simulink model "abEPMAFPLL_compare_sim_c"  (R2020b)
settings: Solver=FixedStepAuto  StartTime=0.0  StopTime=11  FixedStep=Ts  MaxStep=1e-5  RelTol=1e-3
undefined symbols (not defined in the file or in its folder): A_frq_step, A_phase_step, DiscIntNeverNeededParam, f_rad, k_phi, ki, kp, N, t_frq_step, t_phase_step, Ts, V_g, var_noise
libraries: simulink x9, bach_library x3
settings Model: Creator=Martin  LastModifiedBy=Kasper Laustsen
settings DataIOCC: ExternalInput=tt1, tt2, tt3, tt4, tt5, tt6  LoadExternalInput=on
settings SFSimCC: SimCustomHeaderCode=|
  | #include "PLL.h"
  | #include "MAF.h"
settings SFSimCC: SimUserSources=|
  | PLL.c
  | MAF.c

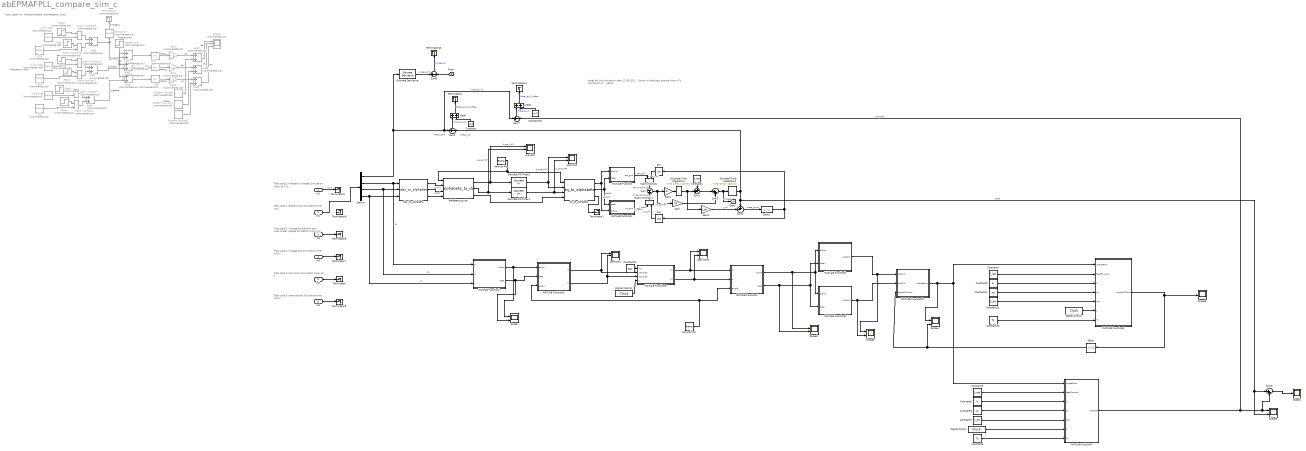
== system abEPMAFPLL_compare_sim_c ==
  note: Input signal incl. noise and phase- and frequency jump
  note: Notes for this simulation
      |
      | date: 22-03-2021,
      | - Solver is fixed step, sample time is Ts (constants.m) - 10kHz
  note: Noise
  note: Phase-jump
  note: theta_grid
  note: theta_pll
  note: Frequency-jump
  note: Test case 2: Phase jumps
      | Simulation time: 70 s
  note: Test case 1: Frequency changes
      | Simulation time: 36.72 s
  note: Test case 3: Voltage fluctuations
      | and over-/under voltage
      | Simulation time: 70 s
  note: Test case 4: Voltage dips
      | Simulation time: 40.9 s
  note: Test case 5: Harmonics
      | Simulation time: 40 s
  note: Test case 6: Interruptions
      | Simulation time: 40.6 s
  In1 : Inport  PortDimensions=4
  In2 : Inport  Port=2  PortDimensions=4
  In3 : Inport  Port=3  PortDimensions=4
  In4 : Inport  Port=4  PortDimensions=4
  In5 : Inport  Port=5  PortDimensions=4
  In6 : Inport  Port=6  PortDimensions=4
  Add{,1..5,7..9} (9 alike) : Sum  Commented=on
  Add11 : Sum
  Add6 : Sum
  Constant : Constant  Value=-pi/2
  Constant1 : Constant  Value=f_rad
  Constant10 : Constant  Value=Ts
  Constant11 : Constant  Value=kp
  Constant12 : Constant  Value=k_phi
  Constant13 : Constant  Value=-pi/2
  Constant24 : Constant  Value=200
  Constant3 : Constant  Value=f_rad
  Constant4 : Constant  Value=f_rad
  Constant5 : Constant  Value=ki
  Constant6 : Constant  Value=kp
  Constant7 : Constant  Value=k_phi
  Constant8 : Constant  Value=Ts
  Constant9 : Constant  Value=ki
  Cos : Trigonometry  Operator=cos
  Delay : Delay  DelayLength=1  SampleTime=Ts
  Delay1 : Delay  DelayLength=1
  Demux : Demux
  Derivative : Derivative  Commented=on
  Digital Clock1 : DigitalClock  SampleTime=Ts
  Digital Clock10 : DigitalClock  SampleTime=Ts
  Digital Clock2 : DigitalClock  SampleTime=Ts
  Discrete Derivative : simulink/Discrete/Discrete Derivative  gainval=1.0  ICPrevScaledInput=0.0  OutMin=[]  OutMax=[]  OutDataType=fixdt(1, 16)  OutScaling=2^-10  DoSatur=off
  Discrete FIR Filter1 : DiscreteFir  Coefficients=[ones(1,N).*1/N]
  Discrete FIR Filter3 : DiscreteFir  Coefficients=[ones(1,N).*1/N]
  Discrete-Time Integrator1 : DiscreteIntegrator  IntegratorMethod=Integration: Trapezoidal  SampleTime=-1  ICPrevOutput=DiscIntNeverNeededParam  ICPrevScaledInput=DiscIntNeverNeededParam
  Discrete-Time Integrator2 : DiscreteIntegrator  IntegratorMethod=Integration: Trapezoidal  SampleTime=-1  ICPrevOutput=DiscIntNeverNeededParam  ICPrevScaledInput=DiscIntNeverNeededParam
  Gain : Gain  Gain=kp
  Gain1 : Gain  Gain=ki
  Gain2 : Gain  Gain=k_phi
  Gain3 : Gain  Commented=on  Gain=V_g
  Gain4 : Gain  Commented=on  Gain=V_g
  Gain5 : Gain  Commented=on  Gain=V_g
  MATLAB Function : MATLAB Function  TreatAsAtomicUnit=on
  MATLAB Function1 : MATLAB Function  TreatAsAtomicUnit=on
  MATLAB Function10 : MATLAB Function  TreatAsAtomicUnit=on
  MATLAB Function2 : MATLAB Function  TreatAsAtomicUnit=on
  MATLAB Function3 : MATLAB Function  TreatAsAtomicUnit=on
  MATLAB Function4 : MATLAB Function  TreatAsAtomicUnit=on
  MATLAB Function5 : MATLAB Function  TreatAsAtomicUnit=on
  MATLAB Function6 : MATLAB Function  TreatAsAtomicUnit=on
  MATLAB Function7 : MATLAB Function  TreatAsAtomicUnit=on
  MATLAB Function8 : MATLAB Function  TreatAsAtomicUnit=on
  MATLAB Function9 : MATLAB Function  TreatAsAtomicUnit=on
  Matrix Multiply : Product
  Matrix Multiply1 : Product
  Matrix Multiply{2..7} (6 alike) : Product  Commented=on
  Random Number : RandomNumber  Commented=on  Variance=var_noise
  Random Number1 : RandomNumber  Commented=on  Variance=var_noise  Seed=1
  Random Number2 : RandomNumber  Commented=on  Variance=var_noise  Seed=2
  Scope{,2..5} (5 alike) : Scope  NumInputPorts=2
  Scope1 : Scope
  Scope6 : Scope
  Sin : Trigonometry
  Sin3 : Trigonometry  Commented=on
  Sin4 : Trigonometry  Commented=on
  Sin5 : Trigonometry  Commented=on
  Step : Step  Commented=on  Time=t_frq_step  Before=1  After=0  SampleTime=0
  Step1 : Step  Commented=on  Time=t_frq_step  SampleTime=0
  Step2 : Step  Commented=on  Time=t_frq_step  Before=1  After=0  SampleTime=0
  Step3 : Step  Commented=on  Time=t_frq_step  SampleTime=0
  Step4 : Step  Commented=on  Time=t_frq_step  Before=1  After=0  SampleTime=0
  Step5 : Step  Commented=on  Time=t_frq_step  SampleTime=0
  Sum : Sum  Inputs=-|+
  Sum1 : Sum  Inputs=++|
  Sum2 : Sum  Inputs=+|-
  Sum3 : Sum  Inputs=|++
  Sum4 : Sum  Inputs=+-|
  Sum6 : Sum  Inputs=+|-
  Sum7 : Sum  Inputs=+|-
  Sum8 : Sum  Inputs=|+-
  Terminator{,1..2,5..11} (10 alike) : Terminator
  Terminator3 : Terminator  Commented=on
  a_frq : simulink/Sources/Ramp  Commented=on  slope=f_rad  start=0  InitialOutput=0
  a_frq_step : simulink/Sources/Ramp  Commented=on  slope=f_rad*A_frq_step  start=t_frq_step  InitialOutput=t_frq_step*f_rad
  abc_to_alphabeta : bach_library/abc_to_alphabeta  SystemSampleTime=-1  VariantActivationTime=update diagram  Latency=0  AutoFrameSizeCalculation=off
  alphabeta_to_dq : bach_library/alphabeta_to_dq  SystemSampleTime=-1  VariantActivationTime=update diagram  Latency=0  AutoFrameSizeCalculation=off
  b_frq : simulink/Sources/Ramp  Commented=on  slope=f_rad  start=0  InitialOutput=-pi*2/3
  b_frq_step : simulink/Sources/Ramp  Commented=on  slope=f_rad*A_frq_step  start=t_frq_step  InitialOutput=t_frq_step*f_rad-pi*2/3
  c_frq : simulink/Sources/Ramp  Commented=on  slope=f_rad  start=0  InitialOutput=pi*2/3
  c_frq_step : simulink/Sources/Ramp  Commented=on  slope=f_rad*A_frq_step  start=t_frq_step  InitialOutput=t_frq_step*f_rad+pi*2/3
  dq_to_alphabeta : bach_library/dq_to_alphabeta  SystemSampleTime=-1  VariantActivationTime=update diagram  Latency=0  AutoFrameSizeCalculation=off
  nominal frq : simulink/Sources/Ramp  slope=f_rad  start=0  InitialOutput=0
  nominal frq1 : simulink/Sources/Ramp  slope=f_rad  start=0  InitialOutput=0
  phase-jump : Step  Commented=on  Time=t_phase_step  After=A_phase_step  SampleTime=0
  phases : Scope  Commented=on  NumInputPorts=3
  post MAF : Scope  NumInputPorts=2
  post MAF1 : Scope  NumInputPorts=2
  pre MAF : Scope  NumInputPorts=3
  pre MAF1 : Scope  NumInputPorts=3
  wires:
  Derivative/1 -> Terminator3/1  "omega_g"
  Step2/1 -> Matrix Multiply2/1
  MATLAB Function/1(cos_grid) -> Matrix Multiply/1  "cos_grid"
  Constant/1 -> Add6/2
  Step/1 -> Matrix Multiply5/1
  Sin5/1 -> Gain5/1  "theta_g"
  Sin3/1 -> Gain3/1  "theta_g"
  Step1/1 -> Matrix Multiply6/1
  a_frq/1 -> Matrix Multiply5/2
  Step4/1 -> Matrix Multiply4/1
  Matrix Multiply2/1 -> Add4/2
  Matrix Multiply7/1 -> Add5/1
  Matrix Multiply6/1 -> Add3/1
  a_frq_step/1 -> Matrix Multiply6/2
  Add6/1 -> Terminator2/1  "theta_err_sim_offset"
  Sum2/1 -> Add6/1  "theta_err_sim"
  Sin/1 -> Matrix Multiply/2  "sin_pll"
  Add1/1 -> Sin4/1
  phase-jump/1 -> Add/1, Add2/1, Add1/1
  Matrix Multiply4/1 -> Add5/2
  Add4/1 -> Add1/2  "b_phase"
  Add9/1 -> phases/3  "pc"
  Add5/1 -> Add2/2  "c_phase"
  Cos/1 -> Matrix Multiply1/2  "cos_pll"
  Add7/1 -> phases/1  "pa"
  Matrix Multiply/1 -> Sum/1  "cos_grid_sin_pll"
  Add8/1 -> phases/2  "pb"
  Add/1 -> Sin3/1
  Random Number/1 -> Add7/2
  Step3/1 -> Matrix Multiply3/1
  Add2/1 -> Sin5/1
  Gain3/1 -> Add7/1  "pa"
  c_frq/1 -> Matrix Multiply4/2
  Matrix Multiply5/1 -> Add3/2
  Add3/1 -> Add/2, Derivative/1  "a_phase"
  Matrix Multiply3/1 -> Add4/1
  Sin4/1 -> Gain4/1  "theta_g"
  MATLAB Function1/1(sin_grid) -> Matrix Multiply1/1  "sin_grid"
  Matrix Multiply1/1 -> Sum/2  "sin_grid_cos_pll"
  Random Number1/1 -> Add8/2
  b_frq_step/1 -> Matrix Multiply3/2
  Random Number2/1 -> Add9/2
  b_frq/1 -> Matrix Multiply2/2
  c_frq_step/1 -> Matrix Multiply7/2
  Gain5/1 -> Add9/1  "pc"
  Gain4/1 -> Add8/1  "pb"
  Step5/1 -> Matrix Multiply7/1
  Gain1/1 -> Discrete-Time Integrator1/1
  Gain/1 -> Sum3/2
  Discrete-Time Integrator1/1 -> Sum1/2, Gain2/1
  Discrete-Time Integrator2/1 -> Scope5/2, Sum8/1, Sum4/1, Sum2/2  "theta"
  Gain2/1 -> Sum4/2  "k_phi"
  Sum4/1 -> Delay1/1  "theta_comp"
  abc_to_alphabeta/3 -> alphabeta_to_dq/4
  dq_to_alphabeta/1 -> MATLAB Function/1(alpha), MATLAB Function1/2(alpha)  "alpha2"
  dq_to_alphabeta/2 -> MATLAB Function1/1(beta), MATLAB Function/2(beta)  "beta2"
  nominal frq/1 -> dq_to_alphabeta/1, alphabeta_to_dq/1
  abc_to_alphabeta/1 -> alphabeta_to_dq/2  "alpha1"
  abc_to_alphabeta/2 -> alphabeta_to_dq/3  "beta1"
  alphabeta_to_dq/2 -> Discrete FIR Filter1/1, pre MAF/2  "q_pre_MAF"
  alphabeta_to_dq/1 -> pre MAF/1, Discrete FIR Filter3/1  "d_pre_MAF"
  Discrete FIR Filter3/1 -> post MAF/1, dq_to_alphabeta/2  "d_post_MAF"
  Discrete FIR Filter1/1 -> post MAF/2, dq_to_alphabeta/3  "q_post_MAF"
  alphabeta_to_dq/3 -> dq_to_alphabeta/4
  Sum1/1 -> Sum3/1
  Constant1/1 -> Sum1/1
  Sum3/1 -> Discrete-Time Integrator2/1, [A]  "omega"
  dq_to_alphabeta/3 -> Terminator1/1
  Demux/1 -> Sum7/1, Sum2/1, Discrete Derivative/1  "thetha_hilb"
  Discrete Derivative/1 -> Sum6/1  "omega_hilb"
  [A] -> Sum6/2
  Sum6/1 -> Terminator10/1  "omega_err"
  In1/1 -> Terminator5/1  "Input"
  In2/1 -> Demux/1
  In3/1 -> Terminator6/1
  In4/1 -> Terminator7/1
  In5/1 -> Terminator/1
  In6/1 -> Terminator8/1
  Sum/1 -> Gain1/1, Gain/1  "sin_grid-pll"
  MATLAB Function9/1(y1) -> post MAF1/1, MATLAB Function4/1(d)
  MATLAB Function9/2(y2) -> post MAF1/2, MATLAB Function4/2(q)
  MATLAB Function3/1(d) -> pre MAF1/1, MATLAB Function9/2(sample1)
  Constant24/1 -> MATLAB Function9/1(len)
  nominal frq1/1 -> MATLAB Function3/3(angle), MATLAB Function4/3(angle)
  MATLAB Function3/2(q) -> pre MAF1/2, MATLAB Function9/3(sample2)
  Delay/1 -> Scope4/2, MATLAB Function10/3(anglePllComp)
  Constant7/1 -> MATLAB Function7/5(kPhi)
  MATLAB Function10/1(phaseError) -> Scope4/1, MATLAB Function7/1(phaseError), MATLAB Function8/1(phaseError)
  MATLAB Function2/1(alpha) -> Scope/1, MATLAB Function3/1(alpha)
  Constant11/1 -> MATLAB Function8/4(kp)
  Constant6/1 -> MATLAB Function7/4(kp)
  Constant9/1 -> MATLAB Function8/3(ki)
  Constant5/1 -> MATLAB Function7/3(ki)
  MATLAB Function8/1(anglePllComp) -> Scope6/1, Delay/1
  Digital Clock2/1 -> MATLAB Function8/6(t)
  Constant10/1 -> MATLAB Function8/7(Ts)
  MATLAB Function7/1(anglePll) -> Sum8/2, Scope5/1, Sum7/2  "anglePll"
  Digital Clock10/1 -> MATLAB Function9/4(t)
  Constant8/1 -> MATLAB Function7/7(Ts)
  MATLAB Function6/1(sinGrid) -> Scope3/2, MATLAB Function10/2(sinGrid)
  Constant4/1 -> MATLAB Function8/2(feedForward)
  Demux/2 -> MATLAB Function2/1(a), abc_to_alphabeta/1  "pa"
  MATLAB Function4/1(alpha) -> Scope2/1, MATLAB Function5/1(alpha), MATLAB Function6/1(alpha)
  Constant12/1 -> MATLAB Function8/5(kPhi)
  Constant3/1 -> MATLAB Function7/2(feedForward)
  Digital Clock1/1 -> MATLAB Function7/6(t)
  MATLAB Function4/2(beta) -> Scope2/2, MATLAB Function5/2(beta), MATLAB Function6/2(beta)
  Demux/4 -> MATLAB Function2/3(c), abc_to_alphabeta/3  "pc"
  Demux/3 -> MATLAB Function2/2(b), abc_to_alphabeta/2  "pb"
  MATLAB Function5/1(cosGrid) -> Scope3/1, MATLAB Function10/1(cosGrid)
  MATLAB Function2/2(beta) -> Scope/2, MATLAB Function3/2(beta)
  Constant13/1 -> Add11/2
  Sum7/1 -> Add11/1  "theta_err_C"
  Add11/1 -> Terminator11/1  "theta_err_C_offset"
  Sum8/1 -> Scope1/1
  Delay1/1 -> Sin/1, Cos/1

== matlab function abEPMAFPLL_compare_sim_c/MATLAB Function10 ==
  data: cosGrid input; phaseError output; sinGrid input; anglePllComp input
function phaseError  = calling_phase_detector(cosGrid, sinGrid, anglePllComp)
% coder.updateBuildInfo('addSourceFiles','abc_to_alphabeta.c');
% coder.cinclude('abc_to_alphabeta.h');
coder.updateBuildInfo('addSourceFiles','PLL.c');
coder.cinclude('PLL.h');

phaseError = 0.0;

phaseError = coder.ceval('phase_detector', cosGrid, sinGrid, anglePllComp);

== matlab function abEPMAFPLL_compare_sim_c/MATLAB Function9 ==
  data: len input; sample1 input; sample2 input; y1 output; t input; y2 output
function [y1, y2] = calling_moving_avg(len, sample1, sample2, t)
% coder.updateBuildInfo('addSourceFiles','moving_avg.c');
% coder.cinclude('moving_avg.h');

coder.updateBuildInfo('addSourceFiles','MAF.c');
coder.cinclude('MAF.h');

y1 = 0.0;
y2 = 0.0;
% y = coder.ceval('moving_avg',u,t);
y1 = coder.ceval('maf1',len, sample1, t);
y2 = coder.ceval('maf2',len, sample2, t);

== matlab function abEPMAFPLL_compare_sim_c/MATLAB Function1 ==
  data: beta input; alpha input; sin_grid output
function sin_grid = sin_grid(beta, alpha)

sin_grid = beta/sqrt(alpha^2+beta^2);

== matlab function abEPMAFPLL_compare_sim_c/MATLAB Function ==
  data: alpha input; cos_grid output; beta input
function cos_grid = cos_grid(alpha, beta)

cos_grid = alpha/sqrt(alpha^2+beta^2);

== matlab function abEPMAFPLL_compare_sim_c/MATLAB Function2 ==
  data: a input; alpha output; b input; c input; beta output
function [alpha,beta] = calling_abc_to_alphabeta(a,b,c)
% coder.updateBuildInfo('addSourceFiles','abc_to_alphabeta.c');
% coder.cinclude('abc_to_alphabeta.h');
coder.updateBuildInfo('addSourceFiles','PLL.c');
coder.cinclude('PLL.h');


alpha = 0.0;
beta = 0.0;

alpha = coder.ceval('abc_to_alpha',a,b,c);
beta = coder.ceval('abc_to_beta',a,b,c);

== matlab function abEPMAFPLL_compare_sim_c/MATLAB Function3 ==
  data: alpha input; d output; beta input; angle input; q output
function [d, q] = calling_alphabeta_to_dq(alpha, beta, angle)
% coder.updateBuildInfo('addSourceFiles','abc_to_alphabeta.c');
% coder.cinclude('abc_to_alphabeta.h');
coder.updateBuildInfo('addSourceFiles','PLL.c');
coder.cinclude('PLL.h');


d = 0.0;
q = 0.0;

d = coder.ceval('alphabeta_to_d',alpha, beta, angle);
q = coder.ceval('alphabeta_to_q',alpha, beta, angle);

== matlab function abEPMAFPLL_compare_sim_c/MATLAB Function4 ==
  data: d input; alpha output; q input; angle input; beta output
function [alpha, beta] = calling_dq_to_alphabeta(d, q, angle)
% coder.updateBuildInfo('addSourceFiles','abc_to_alphabeta.c');
% coder.cinclude('abc_to_alphabeta.h');
coder.updateBuildInfo('addSourceFiles','PLL.c');
coder.cinclude('PLL.h');


alpha = 0.0;
beta = 0.0;

alpha = coder.ceval('dq_to_alpha', d, q, angle);
beta = coder.ceval('dq_to_beta', d, q, angle);

== matlab function abEPMAFPLL_compare_sim_c/MATLAB Function5 ==
  data: alpha input; cosGrid output; beta input
function cosGrid  = calling_cos_grid(alpha, beta)
% coder.updateBuildInfo('addSourceFiles','abc_to_alphabeta.c');
% coder.cinclude('abc_to_alphabeta.h');
coder.updateBuildInfo('addSourceFiles','PLL.c');
coder.cinclude('PLL.h');

cosGrid = 0.0;

cosGrid = coder.ceval('cos_grid', alpha, beta);

== matlab function abEPMAFPLL_compare_sim_c/MATLAB Function6 ==
  data: alpha input; sinGrid output; beta input
function sinGrid  = calling_sin_grid(alpha, beta)
% coder.updateBuildInfo('addSourceFiles','abc_to_alphabeta.c');
% coder.cinclude('abc_to_alphabeta.h');
coder.updateBuildInfo('addSourceFiles','PLL.c');
coder.cinclude('PLL.h');

sinGrid = 0.0;

sinGrid = coder.ceval('sin_grid', alpha, beta);

== matlab function abEPMAFPLL_compare_sim_c/MATLAB Function7 ==
  data: phaseError input; anglePll output; feedForward input; ki input; kp input; kPhi input; t input; Ts input
function anglePll  = calling_pi_regulator(phaseError, feedForward, ki, kp, kPhi, t, Ts)
% coder.updateBuildInfo('addSourceFiles','abc_to_alphabeta.c');
% coder.cinclude('abc_to_alphabeta.h');
coder.updateBuildInfo('addSourceFiles','PLL.c');
coder.cinclude('PLL.h');

anglePll = 0.0;

anglePll = coder.ceval('pi_regulator', phaseError, feedForward, ki, kp, kPhi, t, Ts);

== matlab function abEPMAFPLL_compare_sim_c/MATLAB Function8 ==
  data: phaseError input; anglePllComp output; feedForward input; ki input; kp input; kPhi input; t input; Ts input
function anglePllComp  = calling_pi_regulator_comp(phaseError, feedForward, ki, kp, kPhi, t, Ts)
% coder.updateBuildInfo('addSourceFiles','abc_to_alphabeta.c');
% coder.cinclude('abc_to_alphabeta.h');
coder.updateBuildInfo('addSourceFiles','PLL.c');
coder.cinclude('PLL.h');

anglePllComp = 0.0;

anglePllComp = coder.ceval('pi_regulator_comp', phaseError, feedForward, ki, kp, kPhi, t, Ts);
